simulink model "KalmanFilter"  (R2019a)
settings: Solver=VariableStepAuto  StartTime=0.0  StopTime=10.0  RelTol=1e-3
undefined symbols (not defined in the file): Ad, Bd, C, D, GQG, P0, R, x0
settings Model: Creator=Z634594  LastModifiedBy=Z634594

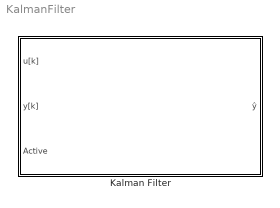
== system KalmanFilter ==
  Kalman Filter : Subsystem
      mask Display: image('C:\Users\Z634594\OneDrive - ZF Friedrichshafen AG\Workspace_MATLAB\14_Tj-Measurement\Simulink\img\Kalman.png');

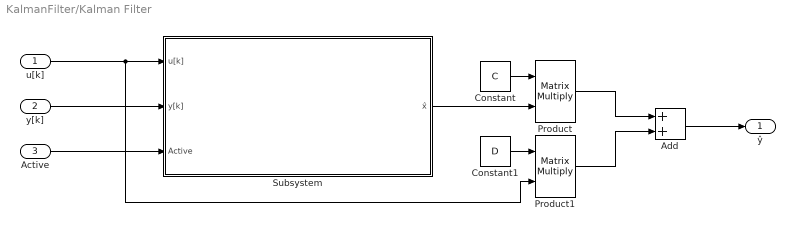
== system KalmanFilter/Kalman Filter ==
  u[k] : Inport
  y[k] : Inport  Port=2
  Active : Inport  Port=3
  Add : Sum
  Constant : Constant  Value=C  VectorParams1D=off
  Constant1 : Constant  Value=D  VectorParams1D=off
  Product : Product  Multiplication=Matrix(*)
  Product1 : Product  Multiplication=Matrix(*)
  Subsystem : Subsystem
      mask Display: image('C:\Users\Z634594\OneDrive - ZF Friedrichshafen AG\Workspace_MATLAB\14_Tj-Measurement\Simulink\img\KalmanEquations.jpg');
  ŷ : Outport
  wires:
  u[k]/1 -> Product1/2, Subsystem/1(u[k])
  y[k]/1 -> Subsystem/2(y[k])
  Constant1/1 -> Product1/1
  Product/1 -> Add/1
  Constant/1 -> Product/1
  Subsystem/1(x̂) -> Product/2
  Add/1 -> ŷ/1
  Product1/1 -> Add/2
  Active/1 -> Subsystem/3(Active)

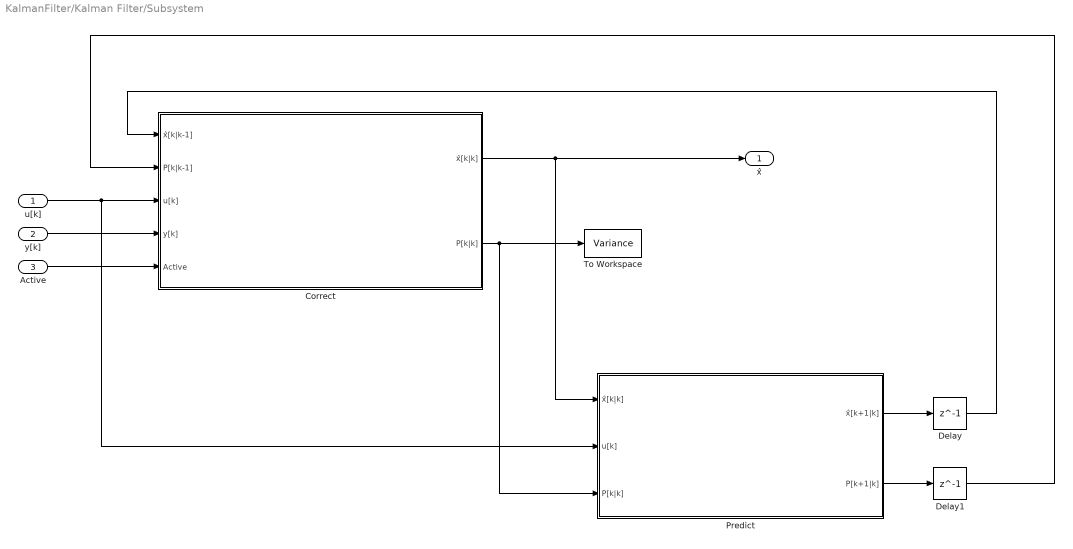
== system KalmanFilter/Kalman Filter/Subsystem ==
  u[k] : Inport
  y[k] : Inport  Port=2
  Active : Inport  Port=3
  Correct : Subsystem
      mask Display: image('C:\Users\Z634594\OneDrive - ZF Friedrichshafen AG\Workspace_MATLAB\14_Tj-Measurement\Simulink\img\Update.png');
  Delay : Delay  DelayLength=1  InitialCondition=x0
  Delay1 : Delay  DelayLength=1  InitialCondition=P0
  Predict : Subsystem
      mask Display: image('C:\Users\Z634594\OneDrive - ZF Friedrichshafen AG\Workspace_MATLAB\14_Tj-Measurement\Simulink\img\Predict.png');
  To Workspace : ToWorkspace  VariableName=Variance  SampleTime=-1
      settings: MaxDataPoints=1
  x̂ : Outport
  wires:
  Predict/1(x̂[k+1|k]) -> Delay/1
  Delay/1 -> Correct/1(x̂[k|k-1])
  Predict/2(P[k+1|k]) -> Delay1/1
  Delay1/1 -> Correct/2(P[k|k-1])
  Correct/1(x̂[k|k]) -> x̂/1, Predict/1(x̂[k|k])
  Correct/2(P[k|k]) -> To Workspace/1, Predict/3(P[k|k])
  u[k]/1 -> Correct/3(u[k]), Predict/2(u[k])
  y[k]/1 -> Correct/4(y[k])
  Active/1 -> Correct/5(Active)

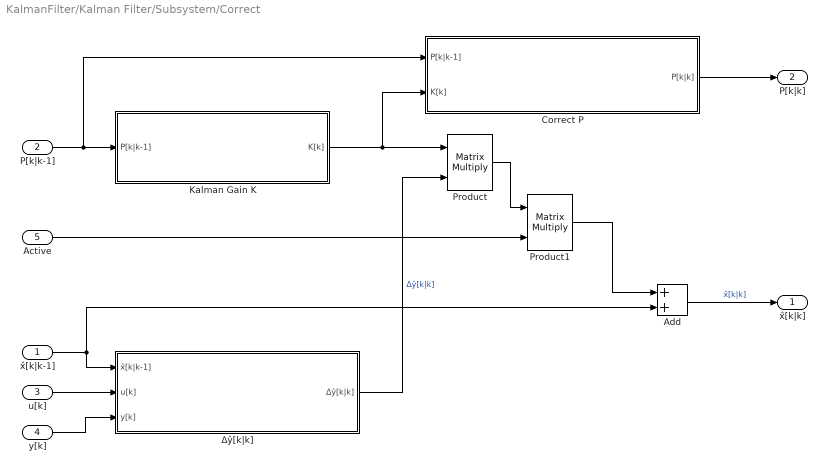
== system KalmanFilter/Kalman Filter/Subsystem/Correct ==
  x̂[k|k-1] : Inport
  P[k|k-1] : Inport  Port=2
  u[k] : Inport  Port=3
  y[k] : Inport  Port=4
  Active : Inport  Port=5
  Add : Sum
  Correct P : Subsystem
      mask Display: image('C:\Users\Z634594\OneDrive - ZF Friedrichshafen AG\Workspace_MATLAB\14_Tj-Measurement\Simulink\img\UpdateP.png');
  Kalman Gain K : Subsystem
      mask Display: image('C:\Users\Z634594\OneDrive - ZF Friedrichshafen AG\Workspace_MATLAB\14_Tj-Measurement\Simulink\img\UpdateK.png');
  Product : Product  Multiplication=Matrix(*)
  Product1 : Product  Multiplication=Matrix(*)
  Δŷ[k|k] : Subsystem
      mask Display: image('C:\Users\Z634594\OneDrive - ZF Friedrichshafen AG\Workspace_MATLAB\14_Tj-Measurement\Simulink\img\CalcdeltaY.png');
  x̂[k|k] : Outport
  P[k|k] : Outport  Port=2
  wires:
  x̂[k|k-1]/1 -> Δŷ[k|k]/1(x̂[k|k-1]), Add/2
  Add/1 -> x̂[k|k]/1  "x̂[k|k]"
  Δŷ[k|k]/1(Δŷ[k|k]) -> Product/2  "Δŷ[k|k]"
  Kalman Gain K/1(K[k]) -> Correct P/2(K[k]), Product/1
  P[k|k-1]/1 -> Correct P/1(P[k|k-1]), Kalman Gain K/1(P[k|k-1])
  Correct P/1(P[k|k]) -> P[k|k]/1
  u[k]/1 -> Δŷ[k|k]/2(u[k])
  y[k]/1 -> Δŷ[k|k]/3(y[k])
  Product/1 -> Product1/1
  Product1/1 -> Add/1
  Active/1 -> Product1/2

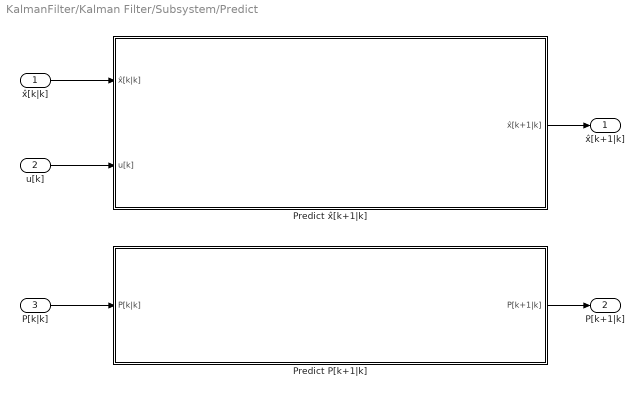
== system KalmanFilter/Kalman Filter/Subsystem/Predict ==
  x̂[k|k] : Inport
  u[k] : Inport  Port=2
  P[k|k] : Inport  Port=3
  Predict P[k+1|k] : Subsystem
      mask Display: image('C:\Users\Z634594\OneDrive - ZF Friedrichshafen AG\Workspace_MATLAB\14_Tj-Measurement\Simulink\img\PredictP.png');
  Predict x̂[k+1|k] : Subsystem
      mask Display: image('C:\Users\Z634594\OneDrive - ZF Friedrichshafen AG\Workspace_MATLAB\14_Tj-Measurement\Simulink\img\Predictx.png');
  x̂[k+1|k] : Outport
  P[k+1|k] : Outport  Port=2
  wires:
  u[k]/1 -> Predict x̂[k+1|k]/2(u[k])
  x̂[k|k]/1 -> Predict x̂[k+1|k]/1(x̂[k|k])
  Predict x̂[k+1|k]/1(x̂[k+1|k]) -> x̂[k+1|k]/1
  Predict P[k+1|k]/1(P[k+1|k]) -> P[k+1|k]/1
  P[k|k]/1 -> Predict P[k+1|k]/1(P[k|k])

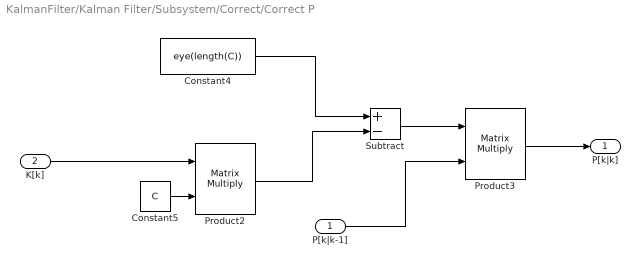
== system KalmanFilter/Kalman Filter/Subsystem/Correct/Correct P ==
  P[k|k-1] : Inport
  K[k] : Inport  Port=2
  Constant4 : Constant  Value=eye(length(C))  VectorParams1D=off
  Constant5 : Constant  Value=C  VectorParams1D=off
  Product2 : Product  Multiplication=Matrix(*)
  Product3 : Product  Multiplication=Matrix(*)
  Subtract : Sum  Inputs=+-
  P[k|k] : Outport
  wires:
  Constant5/1 -> Product2/2
  Constant4/1 -> Subtract/1
  Product2/1 -> Subtract/2
  P[k|k-1]/1 -> Product3/2
  K[k]/1 -> Product2/1
  Subtract/1 -> Product3/1
  Product3/1 -> P[k|k]/1

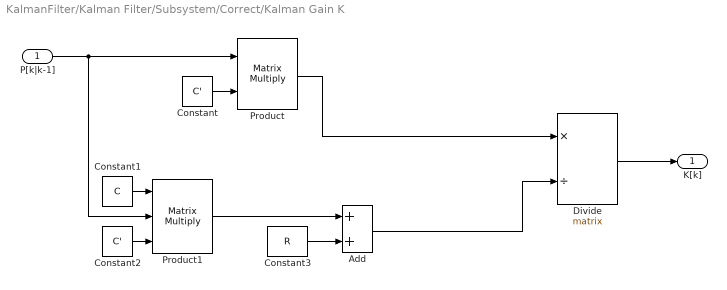
== system KalmanFilter/Kalman Filter/Subsystem/Correct/Kalman Gain K ==
  P[k|k-1] : Inport
  Add : Sum
  Constant : Constant  Value=C'  VectorParams1D=off
  Constant1 : Constant  Value=C  VectorParams1D=off
  Constant2 : Constant  Value=C'  VectorParams1D=off
  Constant3 : Constant  Value=R  VectorParams1D=off
  Divide : Product  Inputs=*/  Multiplication=Matrix(*)
  Product : Product  Multiplication=Matrix(*)
  Product1 : Product  Inputs=3  Multiplication=Matrix(*)
  K[k] : Outport
  wires:
  Constant/1 -> Product/2
  Product/1 -> Divide/1
  Constant1/1 -> Product1/1
  Divide/1 -> K[k]/1
  Constant3/1 -> Add/2
  Add/1 -> Divide/2
  Product1/1 -> Add/1
  P[k|k-1]/1 -> Product1/2, Product/1
  Constant2/1 -> Product1/3

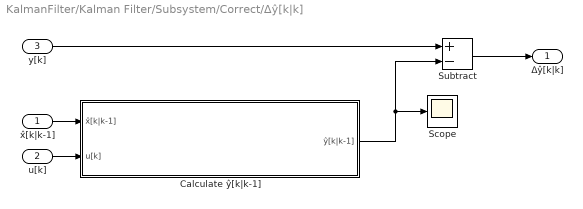
== system KalmanFilter/Kalman Filter/Subsystem/Correct/Δŷ[k|k] ==
  x̂[k|k-1] : Inport
  u[k] : Inport  Port=2
  y[k] : Inport  Port=3
  Calculate ŷ[k|k-1] : Subsystem
      mask Display: image('C:\Users\Z634594\OneDrive - ZF Friedrichshafen AG\Workspace_MATLAB\14_Tj-Measurement\Simulink\img\Calcy.png');
  Scope : Scope
  Subtract : Sum  Inputs=+-
  Δŷ[k|k] : Outport
  wires:
  x̂[k|k-1]/1 -> Calculate ŷ[k|k-1]/1(x̂[k|k-1])
  u[k]/1 -> Calculate ŷ[k|k-1]/2(u[k])
  y[k]/1 -> Subtract/1
  Calculate ŷ[k|k-1]/1(ŷ[k|k-1]) -> Scope/1, Subtract/2
  Subtract/1 -> Δŷ[k|k]/1

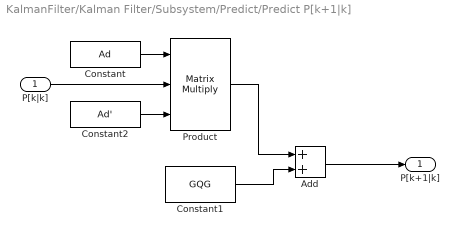
== system KalmanFilter/Kalman Filter/Subsystem/Predict/Predict P[k+1|k] ==
  P[k|k] : Inport
  Add : Sum
  Constant : Constant  Value=Ad  VectorParams1D=off
  Constant1 : Constant  Value=GQG  VectorParams1D=off
  Constant2 : Constant  Value=Ad'  VectorParams1D=off
  Product : Product  Inputs=3  Multiplication=Matrix(*)
  P[k+1|k] : Outport
  wires:
  Constant/1 -> Product/1
  P[k|k]/1 -> Product/2
  Constant2/1 -> Product/3
  Product/1 -> Add/1
  Constant1/1 -> Add/2
  Add/1 -> P[k+1|k]/1

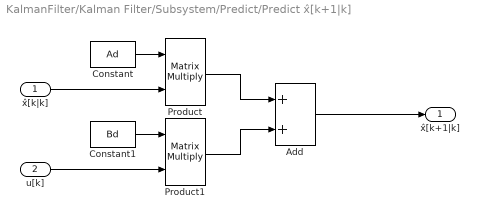
== system KalmanFilter/Kalman Filter/Subsystem/Predict/Predict x̂[k+1|k] ==
  x̂[k|k] : Inport
  u[k] : Inport  Port=2
  Add : Sum
  Constant : Constant  Value=Ad  VectorParams1D=off
  Constant1 : Constant  Value=Bd  VectorParams1D=off
  Product : Product  Multiplication=Matrix(*)
  Product1 : Product  Multiplication=Matrix(*)
  x̂[k+1|k] : Outport
  wires:
  x̂[k|k]/1 -> Product/2
  Add/1 -> x̂[k+1|k]/1
  Constant/1 -> Product/1
  Product/1 -> Add/1
  u[k]/1 -> Product1/2
  Constant1/1 -> Product1/1
  Product1/1 -> Add/2

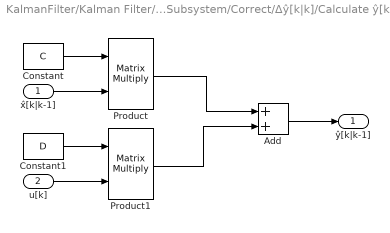
== system KalmanFilter/Kalman Filter/Subsystem/Correct/Δŷ[k|k]/Calculate ŷ[k|k-1] ==
  x̂[k|k-1] : Inport
  u[k] : Inport  Port=2
  Add : Sum
  Constant : Constant  Value=C  VectorParams1D=off
  Constant1 : Constant  Value=D  VectorParams1D=off
  Product : Product  Multiplication=Matrix(*)
  Product1 : Product  Multiplication=Matrix(*)
  ŷ[k|k-1] : Outport
  wires:
  u[k]/1 -> Product1/2
  Product/1 -> Add/1
  x̂[k|k-1]/1 -> Product/2
  Constant/1 -> Product/1
  Constant1/1 -> Product1/1
  Add/1 -> ŷ[k|k-1]/1
  Product1/1 -> Add/2
